simulink model "projekt2"  (R2015a)
settings: Solver=ode3  StartTime=0.0  StopTime=100.0  FixedStep=0.001  RelTol=1e-3
libraries: powerlib_meascontrol x3, simulink_extras x3, sldrtlib x1
settings Model: NumberOfSteps=1000  Creator=Michał  LastModifiedBy=Piotr
settings DebuggingCC: SFNoUnconditionalDefaultTransitionDiag=none

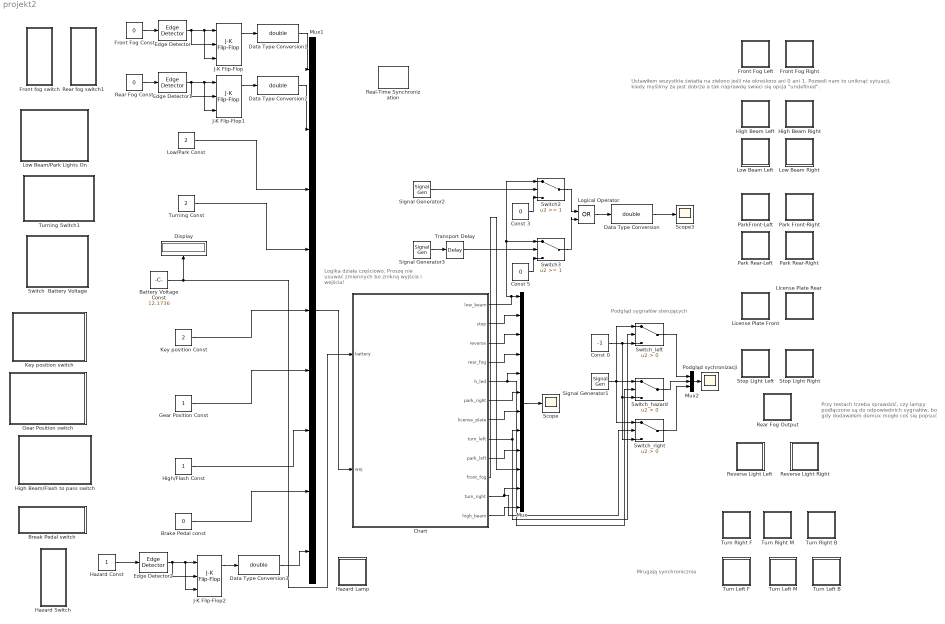
== system projekt2 ==
  note: Mrugają synchronicznie
  note: Przy testach trzeba sprawdzić,
      | czy lampy podłączone są do
      | odpowiednich sygnałów, bo gdy
      | dodawałem demux mogło coś się popsuć
  note: Logika działa częściowo.
      | Proszę nie usuwać zmiennych bo
      |  znikną wyjścia i wejścia!
  note: Podgląd sygnałów sterujących
  note: Ustawiłem wszystkie światła na zielono jeśli nie określono ani 0 ani 1.
      | Pozwoli nam to uniknąć sytuacji, kiedy myślimy że jest dobrze a tak naprawdę swieci się opcja "undefined".
  Battery Voltage Const : Constant  Value=12.1736
  Brake Pedal const : Constant  Value=0
  Break Pedal switch : Subsystem  DialogController=hmiCreateDDGDialog  IsWebBlock=on  mask(MathWorksWebBlock){webBlockId=9203b425-6a6c-4a56-bfc7-19389e98b110, webBlockType=sliderswitch, ShowInLibBrowser=on, ShowInitialText=on, HMISrcModelName=projekt2_bro}
      mask prompts: webBlockId "WebBlock Id"; webBlockType "WebBlock Type"; HMISrcModelName "Source Model"
      mask Help: helpview([docroot '/mapfiles/simulink.map'], 'hmi_slider_switch')
      mask Display:
      | if strcmp(get_param(bdroot(gcb),'BlockDiagramType'), 'library')
      |     image([(matlabroot) '/toolbox/simulink/hmi/icons/SliderSwitch.png']);
      | end
  Chart : Stateflow chart  TreatAsAtomicUnit=on
  Const 0 : Constant  Value=-1
  Const 3 : Constant  Value=0
  Const 5 : Constant  Value=0
  Data Type Conversion{,1..3} (4 alike) : DataTypeConversion  OutDataTypeStr=double
  Display : Display
  Edge Detector : powerlib_meascontrol/Logic/Edge Detector  model=Rising  ic=0  Ts=0
  Edge Detector1 : powerlib_meascontrol/Logic/Edge Detector  model=Rising  ic=0  Ts=0
  Edge Detector2 : powerlib_meascontrol/Logic/Edge Detector  model=Rising  ic=0  Ts=0
  Front Fog Const : Constant  Value=0
  Front Fog Left : Subsystem  DialogController=hmiCreateDDGDialog  IsWebBlock=on  mask(MathWorksWebBlock){webBlockId=1137b8ce-eb4e-40f8-b4a0-8fd8244cb3ae, webBlockType=lamp, ShowInLibBrowser=on, ShowInitialText=on, HMISrcModelName=projekt2_bro}
      mask prompts: webBlockType "WebBlock Type"; HMISrcModelName "Source Model"
      mask Help: helpview([docroot '/mapfiles/simulink.map'], 'hmi_lamp')
      mask Display:
      | if strcmp(get_param(bdroot(gcb),'BlockDiagramType'), 'library')
      |     image([(matlabroot) '/toolbox/simulink/hmi/icons/Lamp.png']);
      | end
  Front Fog Right : Subsystem  DialogController=hmiCreateDDGDialog  IsWebBlock=on  mask(MathWorksWebBlock){webBlockId=91a87ca5-cdac-4de7-a024-86dcea0ba100, webBlockType=lamp, ShowInLibBrowser=on, ShowInitialText=on, HMISrcModelName=projekt2_bro}
      mask prompts: webBlockType "WebBlock Type"; HMISrcModelName "Source Model"
      mask Help: helpview([docroot '/mapfiles/simulink.map'], 'hmi_lamp')
      mask Display:
      | if strcmp(get_param(bdroot(gcb),'BlockDiagramType'), 'library')
      |     image([(matlabroot) '/toolbox/simulink/hmi/icons/Lamp.png']);
      | end
  Front fog switch : Subsystem  DialogController=hmiCreateDDGDialog  IsWebBlock=on  mask(MathWorksWebBlock){webBlockId=82ea03f9-1116-4696-a3c0-68725e62bad1, webBlockType=toggleswitch, ShowInLibBrowser=on, ShowInitialText=on, HMISrcModelName=projekt2_bro}
      mask prompts: webBlockId "WebBlock Id"; webBlockType "WebBlock Type"; HMISrcModelName "Source Model"
      mask Help: helpview([docroot '/mapfiles/simulink.map'], 'hmi_toggle_switch')
      mask Display:
      | if strcmp(get_param(bdroot(gcb),'BlockDiagramType'), 'library')
      |     image([(matlabroot) '/toolbox/simulink/hmi/icons/ToggleSwitch.png']);
      | end
  Gear Position Const : Constant
  Gear Position switch : Subsystem  DialogController=hmiCreateDDGDialog  IsWebBlock=on  mask(MathWorksWebBlock){webBlockId=9873bca9-f904-40ed-a9f4-ca11686aee94, webBlockType=discreteknob, ShowInLibBrowser=on, ShowInitialText=on, HMISrcModelName=projekt2_bro}
      mask prompts: webBlockId "WebBlock Id"; webBlockType "WebBlock Type"; HMISrcModelName "Source Model"
      mask Help: helpview([docroot '/mapfiles/simulink.map'], 'hmi_rotary_switch')
      mask Display:
      | model = bdroot(gcb);
      | if strcmp(get_param(model,'BlockDiagramType'), 'library')
      |     image([(matlabroot) '/toolbox/simulink/hmi/icons/DiscreteKnob.png']);
      | end
  Hazard Const : Constant
  Hazard Lamp : Subsystem  DialogController=hmiCreateDDGDialog  IsWebBlock=on  mask(MathWorksWebBlock){webBlockId=bb1142b6-d357-4f8e-bbaa-be8425e77c63, webBlockType=lamp, ShowInLibBrowser=on, ShowInitialText=on, HMISrcModelName=projekt2_bro}
      mask prompts: webBlockType "WebBlock Type"; HMISrcModelName "Source Model"
      mask Help: helpview([docroot '/mapfiles/simulink.map'], 'hmi_lamp')
      mask Display:
      | if strcmp(get_param(bdroot(gcb),'BlockDiagramType'), 'library')
      |     image([(matlabroot) '/toolbox/simulink/hmi/icons/Lamp.png']);
      | end
  Hazard Switch : Subsystem  DialogController=hmiCreateDDGDialog  IsWebBlock=on  mask(MathWorksWebBlock){webBlockId=797843e7-9493-43d7-b5ed-a5b1ec2f2620, webBlockType=toggleswitch, ShowInLibBrowser=on, ShowInitialText=on, HMISrcModelName=projekt2_bro}
      mask prompts: webBlockId "WebBlock Id"; webBlockType "WebBlock Type"; HMISrcModelName "Source Model"
      mask Help: helpview([docroot '/mapfiles/simulink.map'], 'hmi_toggle_switch')
      mask Display:
      | if strcmp(get_param(bdroot(gcb),'BlockDiagramType'), 'library')
      |     image([(matlabroot) '/toolbox/simulink/hmi/icons/ToggleSwitch.png']);
      | end
  High Beam Left : Subsystem  DialogController=hmiCreateDDGDialog  IsWebBlock=on  mask(MathWorksWebBlock){webBlockId=ca8d7307-15bb-4202-84d0-933cf6b75606, webBlockType=lamp, ShowInLibBrowser=on, ShowInitialText=on, HMISrcModelName=projekt2_bro}
      mask prompts: webBlockType "WebBlock Type"; HMISrcModelName "Source Model"
      mask Help: helpview([docroot '/mapfiles/simulink.map'], 'hmi_lamp')
      mask Display:
      | if strcmp(get_param(bdroot(gcb),'BlockDiagramType'), 'library')
      |     image([(matlabroot) '/toolbox/simulink/hmi/icons/Lamp.png']);
      | end
  High Beam Right : Subsystem  DialogController=hmiCreateDDGDialog  IsWebBlock=on  mask(MathWorksWebBlock){webBlockId=1f4769ad-4ae1-430d-b7b3-b710370c0a18, webBlockType=lamp, ShowInLibBrowser=on, ShowInitialText=on, HMISrcModelName=projekt2_bro}
      mask prompts: webBlockType "WebBlock Type"; HMISrcModelName "Source Model"
      mask Help: helpview([docroot '/mapfiles/simulink.map'], 'hmi_lamp')
      mask Display:
      | if strcmp(get_param(bdroot(gcb),'BlockDiagramType'), 'library')
      |     image([(matlabroot) '/toolbox/simulink/hmi/icons/Lamp.png']);
      | end
  High Beam/Flash to pass switch : Subsystem  DialogController=hmiCreateDDGDialog  IsWebBlock=on  mask(MathWorksWebBlock){webBlockId=cb76618a-e943-4ab4-b6d9-c65f6536b605, webBlockType=discreteknob, ShowInLibBrowser=on, ShowInitialText=on, HMISrcModelName=projekt2_bro}
      mask prompts: webBlockId "WebBlock Id"; webBlockType "WebBlock Type"; HMISrcModelName "Source Model"
      mask Help: helpview([docroot '/mapfiles/simulink.map'], 'hmi_rotary_switch')
      mask Display:
      | model = bdroot(gcb);
      | if strcmp(get_param(model,'BlockDiagramType'), 'library')
      |     image([(matlabroot) '/toolbox/simulink/hmi/icons/DiscreteKnob.png']);
      | end
  High/Flash Const : Constant
  J-K Flip-Flop : simulink_extras/Flip Flops/J-K Flip-Flop  initial_condition=0
  J-K Flip-Flop1 : simulink_extras/Flip Flops/J-K Flip-Flop  initial_condition=0
  J-K Flip-Flop2 : simulink_extras/Flip Flops/J-K Flip-Flop  initial_condition=0
  Key position Const : Constant  Value=2
  Key position switch : Subsystem  DialogController=hmiCreateDDGDialog  IsWebBlock=on  mask(MathWorksWebBlock){webBlockId=6a93fa06-9241-43a4-9533-b6adabf72aa1, webBlockType=discreteknob, ShowInLibBrowser=on, ShowInitialText=on, HMISrcModelName=projekt2_bro}
      mask prompts: webBlockId "WebBlock Id"; webBlockType "WebBlock Type"; HMISrcModelName "Source Model"
      mask Help: helpview([docroot '/mapfiles/simulink.map'], 'hmi_rotary_switch')
      mask Display:
      | model = bdroot(gcb);
      | if strcmp(get_param(model,'BlockDiagramType'), 'library')
      |     image([(matlabroot) '/toolbox/simulink/hmi/icons/DiscreteKnob.png']);
      | end
  License Plate Front : Subsystem  DialogController=hmiCreateDDGDialog  IsWebBlock=on  mask(MathWorksWebBlock){webBlockId=33e809d7-7293-40ab-82d3-89bf48253b8e, webBlockType=lamp, ShowInLibBrowser=on, ShowInitialText=on, HMISrcModelName=projekt2_bro}
      mask prompts: webBlockType "WebBlock Type"; HMISrcModelName "Source Model"
      mask Help: helpview([docroot '/mapfiles/simulink.map'], 'hmi_lamp')
      mask Display:
      | if strcmp(get_param(bdroot(gcb),'BlockDiagramType'), 'library')
      |     image([(matlabroot) '/toolbox/simulink/hmi/icons/Lamp.png']);
      | end
  License Plate Rear : Subsystem  DialogController=hmiCreateDDGDialog  IsWebBlock=on  mask(MathWorksWebBlock){webBlockId=e2d37614-ade8-4960-9755-81aca5d14707, webBlockType=lamp, ShowInLibBrowser=on, ShowInitialText=on, HMISrcModelName=projekt2_bro}
      mask prompts: webBlockType "WebBlock Type"; HMISrcModelName "Source Model"
      mask Help: helpview([docroot '/mapfiles/simulink.map'], 'hmi_lamp')
      mask Display:
      | if strcmp(get_param(bdroot(gcb),'BlockDiagramType'), 'library')
      |     image([(matlabroot) '/toolbox/simulink/hmi/icons/Lamp.png']);
      | end
  Logical Operator : Logic  Operator=OR  IconShape=distinctive  AllPortsSameDT=off  OutDataTypeStr=boolean
  Low Beam Left : Subsystem  DialogController=hmiCreateDDGDialog  IsWebBlock=on  mask(MathWorksWebBlock){webBlockId=93f46513-60d2-4d66-bc1a-d0f0cd962895, webBlockType=lamp, ShowInLibBrowser=on, ShowInitialText=on, HMISrcModelName=projekt2_bro}
      mask prompts: webBlockType "WebBlock Type"; HMISrcModelName "Source Model"
      mask Help: helpview([docroot '/mapfiles/simulink.map'], 'hmi_lamp')
      mask Display:
      | if strcmp(get_param(bdroot(gcb),'BlockDiagramType'), 'library')
      |     image([(matlabroot) '/toolbox/simulink/hmi/icons/Lamp.png']);
      | end
  Low Beam Right : Subsystem  DialogController=hmiCreateDDGDialog  IsWebBlock=on  mask(MathWorksWebBlock){webBlockId=cbd13759-b6c8-48cc-8b95-5d08102353a4, webBlockType=lamp, ShowInLibBrowser=on, ShowInitialText=on, HMISrcModelName=projekt2_bro}
      mask prompts: webBlockType "WebBlock Type"; HMISrcModelName "Source Model"
      mask Help: helpview([docroot '/mapfiles/simulink.map'], 'hmi_lamp')
      mask Display:
      | if strcmp(get_param(bdroot(gcb),'BlockDiagramType'), 'library')
      |     image([(matlabroot) '/toolbox/simulink/hmi/icons/Lamp.png']);
      | end
  Low Beam/Park Lights On : Subsystem  DialogController=hmiCreateDDGDialog  IsWebBlock=on  mask(MathWorksWebBlock){webBlockId=c2ad75a2-8b3b-4bc8-8975-68c2dc12f70e, webBlockType=discreteknob, ShowInLibBrowser=on, ShowInitialText=on, HMISrcModelName=projekt2_bro}
      mask prompts: webBlockId "WebBlock Id"; webBlockType "WebBlock Type"; HMISrcModelName "Source Model"
      mask Help: helpview([docroot '/mapfiles/simulink.map'], 'hmi_rotary_switch')
      mask Display:
      | model = bdroot(gcb);
      | if strcmp(get_param(model,'BlockDiagramType'), 'library')
      |     image([(matlabroot) '/toolbox/simulink/hmi/icons/DiscreteKnob.png']);
      | end
  Low/Park Const : Constant  Value=2
  Mux : Mux  Inputs=12
  Mux1 : Mux  Inputs=9
  Mux2 : Mux  Inputs=3
  Park Front-Right : Subsystem  DialogController=hmiCreateDDGDialog  IsWebBlock=on  mask(MathWorksWebBlock){webBlockId=9b7f9617-a09f-4c99-8fef-94e297c97476, webBlockType=lamp, ShowInLibBrowser=on, ShowInitialText=on, HMISrcModelName=projekt2_bro}
      mask prompts: webBlockType "WebBlock Type"; HMISrcModelName "Source Model"
      mask Help: helpview([docroot '/mapfiles/simulink.map'], 'hmi_lamp')
      mask Display:
      | if strcmp(get_param(bdroot(gcb),'BlockDiagramType'), 'library')
      |     image([(matlabroot) '/toolbox/simulink/hmi/icons/Lamp.png']);
      | end
  Park Rear-Left : Subsystem  DialogController=hmiCreateDDGDialog  IsWebBlock=on  mask(MathWorksWebBlock){webBlockId=f0d072a0-1d13-4b2c-9055-2934ad2aeeda, webBlockType=lamp, ShowInLibBrowser=on, ShowInitialText=on, HMISrcModelName=projekt2_bro}
      mask prompts: webBlockType "WebBlock Type"; HMISrcModelName "Source Model"
      mask Help: helpview([docroot '/mapfiles/simulink.map'], 'hmi_lamp')
      mask Display:
      | if strcmp(get_param(bdroot(gcb),'BlockDiagramType'), 'library')
      |     image([(matlabroot) '/toolbox/simulink/hmi/icons/Lamp.png']);
      | end
  Park Rear-Right : Subsystem  DialogController=hmiCreateDDGDialog  IsWebBlock=on  mask(MathWorksWebBlock){webBlockId=6a2c4c4f-cbef-489d-a936-82416b980595, webBlockType=lamp, ShowInLibBrowser=on, ShowInitialText=on, HMISrcModelName=projekt2_bro}
      mask prompts: webBlockType "WebBlock Type"; HMISrcModelName "Source Model"
      mask Help: helpview([docroot '/mapfiles/simulink.map'], 'hmi_lamp')
      mask Display:
      | if strcmp(get_param(bdroot(gcb),'BlockDiagramType'), 'library')
      |     image([(matlabroot) '/toolbox/simulink/hmi/icons/Lamp.png']);
      | end
  ParkFront-Left : Subsystem  DialogController=hmiCreateDDGDialog  IsWebBlock=on  mask(MathWorksWebBlock){webBlockId=2a1e2c86-b327-4131-a799-a6f04c855dbb, webBlockType=lamp, ShowInLibBrowser=on, ShowInitialText=on, HMISrcModelName=projekt2_bro}
      mask prompts: webBlockType "WebBlock Type"; HMISrcModelName "Source Model"
      mask Help: helpview([docroot '/mapfiles/simulink.map'], 'hmi_lamp')
      mask Display:
      | if strcmp(get_param(bdroot(gcb),'BlockDiagramType'), 'library')
      |     image([(matlabroot) '/toolbox/simulink/hmi/icons/Lamp.png']);
      | end
  Podgląd sychronizacji : Scope
  Real-Time Synchronization : sldrtlib/Real-Time Synchronization  SampleTime=0.1  MaxMissedTicks=10  ShowMissedTicks=off  YieldWhenWaiting=off
  Rear Fog Const : Constant  Value=0
  Rear Fog Output : Subsystem  DialogController=hmiCreateDDGDialog  IsWebBlock=on  mask(MathWorksWebBlock){webBlockId=c86d492b-d5b5-45fd-8d57-4ca5ff4cc7e3, webBlockType=lamp, ShowInLibBrowser=on, ShowInitialText=on, HMISrcModelName=projekt2_bro}
      mask prompts: webBlockType "WebBlock Type"; HMISrcModelName "Source Model"
      mask Help: helpview([docroot '/mapfiles/simulink.map'], 'hmi_lamp')
      mask Display:
      | if strcmp(get_param(bdroot(gcb),'BlockDiagramType'), 'library')
      |     image([(matlabroot) '/toolbox/simulink/hmi/icons/Lamp.png']);
      | end
  Rear fog switch1 : Subsystem  DialogController=hmiCreateDDGDialog  IsWebBlock=on  mask(MathWorksWebBlock){webBlockId=a6fd6b9e-e7fc-4e66-962f-fca6c1e6a3ec, webBlockType=toggleswitch, ShowInLibBrowser=on, ShowInitialText=on, HMISrcModelName=projekt2_bro}
      mask prompts: webBlockId "WebBlock Id"; webBlockType "WebBlock Type"; HMISrcModelName "Source Model"
      mask Help: helpview([docroot '/mapfiles/simulink.map'], 'hmi_toggle_switch')
      mask Display:
      | if strcmp(get_param(bdroot(gcb),'BlockDiagramType'), 'library')
      |     image([(matlabroot) '/toolbox/simulink/hmi/icons/ToggleSwitch.png']);
      | end
  Reverse Light Left : Subsystem  DialogController=hmiCreateDDGDialog  IsWebBlock=on  mask(MathWorksWebBlock){webBlockId=1216e6e6-a2b0-45d0-bfe3-2d719345f04b, webBlockType=lamp, ShowInLibBrowser=on, ShowInitialText=on, HMISrcModelName=projekt2_bro}
      mask prompts: webBlockType "WebBlock Type"; HMISrcModelName "Source Model"
      mask Help: helpview([docroot '/mapfiles/simulink.map'], 'hmi_lamp')
      mask Display:
      | if strcmp(get_param(bdroot(gcb),'BlockDiagramType'), 'library')
      |     image([(matlabroot) '/toolbox/simulink/hmi/icons/Lamp.png']);
      | end
  Reverse Light Right : Subsystem  DialogController=hmiCreateDDGDialog  IsWebBlock=on  mask(MathWorksWebBlock){webBlockId=aab8cf70-1b34-41c4-b955-76454d5b273c, webBlockType=lamp, ShowInLibBrowser=on, ShowInitialText=on, HMISrcModelName=projekt2_bro}
      mask prompts: webBlockType "WebBlock Type"; HMISrcModelName "Source Model"
      mask Help: helpview([docroot '/mapfiles/simulink.map'], 'hmi_lamp')
      mask Display:
      | if strcmp(get_param(bdroot(gcb),'BlockDiagramType'), 'library')
      |     image([(matlabroot) '/toolbox/simulink/hmi/icons/Lamp.png']);
      | end
  Scope : Scope
  Scope3 : Scope
      settings: SaveName=ScopeData3
  Signal Generator1 : SignalGenerator  WaveForm=square  Frequency=1.5
  Signal Generator2 : SignalGenerator  WaveForm=square  Frequency=100
  Signal Generator3 : SignalGenerator  WaveForm=square  Frequency=100
  Stop Light Left : Subsystem  DialogController=hmiCreateDDGDialog  IsWebBlock=on  mask(MathWorksWebBlock){webBlockId=fe2cd1c8-1e5b-41df-9169-199d59002129, webBlockType=lamp, ShowInLibBrowser=on, ShowInitialText=on, HMISrcModelName=projekt2_bro}
      mask prompts: webBlockType "WebBlock Type"; HMISrcModelName "Source Model"
      mask Help: helpview([docroot '/mapfiles/simulink.map'], 'hmi_lamp')
      mask Display:
      | if strcmp(get_param(bdroot(gcb),'BlockDiagramType'), 'library')
      |     image([(matlabroot) '/toolbox/simulink/hmi/icons/Lamp.png']);
      | end
  Stop Light Right : Subsystem  DialogController=hmiCreateDDGDialog  IsWebBlock=on  mask(MathWorksWebBlock){webBlockId=e28d537a-d055-4b98-9d36-b585e9c6a455, webBlockType=lamp, ShowInLibBrowser=on, ShowInitialText=on, HMISrcModelName=projekt2_bro}
      mask prompts: webBlockType "WebBlock Type"; HMISrcModelName "Source Model"
      mask Help: helpview([docroot '/mapfiles/simulink.map'], 'hmi_lamp')
      mask Display:
      | if strcmp(get_param(bdroot(gcb),'BlockDiagramType'), 'library')
      |     image([(matlabroot) '/toolbox/simulink/hmi/icons/Lamp.png']);
      | end
  Switch  Battery Voltage : Subsystem  DialogController=hmiCreateDDGDialog  IsWebBlock=on  mask(MathWorksWebBlock){webBlockId=9fcb4338-6d0a-49e3-9d35-1b064d171cad, webBlockType=continuousknob, ShowInLibBrowser=on, ShowInitialText=on, HMISrcModelName=projekt2_bro}
      mask prompts: webBlockId "WebBlock Id"; webBlockType "WebBlock Type"; HMISrcModelName "Source Model"
      mask Help: helpview([docroot '/mapfiles/simulink.map'], 'hmi_knob')
      mask Display:
      | if strcmp(get_param(bdroot(gcb),'BlockDiagramType'), 'library')
      |     image([(matlabroot) '/toolbox/simulink/hmi/icons/ContinuousKnob.png']);
      | end
  Switch2 : Switch  Threshold=1
  Switch3 : Switch  Threshold=1
  Switch_hazard : Switch  Criteria=u2 > Threshold
  Switch_left : Switch  Criteria=u2 > Threshold
  Switch_right : Switch  Criteria=u2 > Threshold
  Transport Delay : TransportDelay  DelayTime=0.004
  Turn Left B : Subsystem  DialogController=hmiCreateDDGDialog  IsWebBlock=on  mask(MathWorksWebBlock){webBlockId=4dada64b-7e7a-4b74-8d0d-b8c062fae480, webBlockType=lamp, ShowInLibBrowser=on, ShowInitialText=on, HMISrcModelName=projekt2_bro}
      mask prompts: webBlockType "WebBlock Type"; HMISrcModelName "Source Model"
      mask Help: helpview([docroot '/mapfiles/simulink.map'], 'hmi_lamp')
      mask Display:
      | if strcmp(get_param(bdroot(gcb),'BlockDiagramType'), 'library')
      |     image([(matlabroot) '/toolbox/simulink/hmi/icons/Lamp.png']);
      | end
  Turn Left F : Subsystem  DialogController=hmiCreateDDGDialog  IsWebBlock=on  mask(MathWorksWebBlock){webBlockId=e6f60506-cdc4-4a96-ad0a-e579d3159bd8, webBlockType=lamp, ShowInLibBrowser=on, ShowInitialText=on, HMISrcModelName=projekt2_bro}
      mask prompts: webBlockType "WebBlock Type"; HMISrcModelName "Source Model"
      mask Help: helpview([docroot '/mapfiles/simulink.map'], 'hmi_lamp')
      mask Display:
      | if strcmp(get_param(bdroot(gcb),'BlockDiagramType'), 'library')
      |     image([(matlabroot) '/toolbox/simulink/hmi/icons/Lamp.png']);
      | end
  Turn Left M : Subsystem  DialogController=hmiCreateDDGDialog  IsWebBlock=on  mask(MathWorksWebBlock){webBlockId=86cbbfda-27e6-47d5-9477-a59dd7b37ef2, webBlockType=lamp, ShowInLibBrowser=on, ShowInitialText=on, HMISrcModelName=projekt2_bro}
      mask prompts: webBlockType "WebBlock Type"; HMISrcModelName "Source Model"
      mask Help: helpview([docroot '/mapfiles/simulink.map'], 'hmi_lamp')
      mask Display:
      | if strcmp(get_param(bdroot(gcb),'BlockDiagramType'), 'library')
      |     image([(matlabroot) '/toolbox/simulink/hmi/icons/Lamp.png']);
      | end
  Turn Right B : Subsystem  DialogController=hmiCreateDDGDialog  IsWebBlock=on  mask(MathWorksWebBlock){webBlockId=de10194a-7102-4529-bffa-3ba9fd236063, webBlockType=lamp, ShowInLibBrowser=on, ShowInitialText=on, HMISrcModelName=projekt2_bro}
      mask prompts: webBlockType "WebBlock Type"; HMISrcModelName "Source Model"
      mask Help: helpview([docroot '/mapfiles/simulink.map'], 'hmi_lamp')
      mask Display:
      | if strcmp(get_param(bdroot(gcb),'BlockDiagramType'), 'library')
      |     image([(matlabroot) '/toolbox/simulink/hmi/icons/Lamp.png']);
      | end
  Turn Right F : Subsystem  DialogController=hmiCreateDDGDialog  IsWebBlock=on  mask(MathWorksWebBlock){webBlockId=8d34aea4-920d-4358-901e-989a77b658ef, webBlockType=lamp, ShowInLibBrowser=on, ShowInitialText=on, HMISrcModelName=projekt2_bro}
      mask prompts: webBlockType "WebBlock Type"; HMISrcModelName "Source Model"
      mask Help: helpview([docroot '/mapfiles/simulink.map'], 'hmi_lamp')
      mask Display:
      | if strcmp(get_param(bdroot(gcb),'BlockDiagramType'), 'library')
      |     image([(matlabroot) '/toolbox/simulink/hmi/icons/Lamp.png']);
      | end
  Turn Right M : Subsystem  DialogController=hmiCreateDDGDialog  IsWebBlock=on  mask(MathWorksWebBlock){webBlockId=1d267936-957d-42ac-8213-13ca1cae1405, webBlockType=lamp, ShowInLibBrowser=on, ShowInitialText=on, HMISrcModelName=projekt2_bro}
      mask prompts: webBlockType "WebBlock Type"; HMISrcModelName "Source Model"
      mask Help: helpview([docroot '/mapfiles/simulink.map'], 'hmi_lamp')
      mask Display:
      | if strcmp(get_param(bdroot(gcb),'BlockDiagramType'), 'library')
      |     image([(matlabroot) '/toolbox/simulink/hmi/icons/Lamp.png']);
      | end
  Turning Const : Constant  Value=2
  Turning Switch1 : Subsystem  DialogController=hmiCreateDDGDialog  IsWebBlock=on  mask(MathWorksWebBlock){webBlockId=0fc1dd6b-b7af-4fe7-8c63-8dd4046cb8f2, webBlockType=discreteknob, ShowInLibBrowser=on, ShowInitialText=on, HMISrcModelName=projekt2_bro}
      mask prompts: webBlockId "WebBlock Id"; webBlockType "WebBlock Type"; HMISrcModelName "Source Model"
      mask Help: helpview([docroot '/mapfiles/simulink.map'], 'hmi_rotary_switch')
      mask Display:
      | model = bdroot(gcb);
      | if strcmp(get_param(model,'BlockDiagramType'), 'library')
      |     image([(matlabroot) '/toolbox/simulink/hmi/icons/DiscreteKnob.png']);
      | end
  wires:
  Battery Voltage Const/1 -> Chart/1(battery), Display/1
  Chart/1(low_beam) -> Mux/1, Switch3/1, Switch2/1
  Chart/2(stop) -> Mux/2
  Chart/3(reverse) -> Mux/3
  Chart/4(rear_fog) -> Mux/4
  Chart/6(park_right) -> Mux/6
  Chart/8(turn_left) -> Mux/8, Switch_left/2
  Chart/9(park_left) -> Mux/9
  Chart/10(front_fog) -> Mux/10
  Chart/12(high_beam) -> Mux/12
  Mux/1 -> Scope/1
  Chart/5(h_led) -> Switch_hazard/2, Mux/5
  Low/Park Const/1 -> Mux1/3
  Turning Const/1 -> Mux1/4
  Key position Const/1 -> Mux1/5
  Gear Position Const/1 -> Mux1/6
  High/Flash Const/1 -> Mux1/7
  Brake Pedal const/1 -> Mux1/8
  Mux1/1 -> Chart/2(wej)
  Chart/7(license_plate) -> Mux/7
  Chart/11(turn_right) -> Mux/11, Switch_right/2
  Switch_left/1 -> Mux2/1
  Const 0/1 -> Switch_right/3, Switch_hazard/3, Switch_left/3
  Switch_right/1 -> Mux2/3
  Signal Generator1/1 -> Switch_hazard/1, Switch_right/1, Switch_left/1
  Signal Generator3/1 -> Transport Delay/1
  Data Type Conversion/1 -> Scope3/1
  Signal Generator2/1 -> Switch2/2
  Const 3/1 -> Switch2/3
  Transport Delay/1 -> Switch3/2
  Const 5/1 -> Switch3/3
  Switch3/1 -> Logical Operator/2
  Switch2/1 -> Logical Operator/1
  Logical Operator/1 -> Data Type Conversion/1
  Switch_hazard/1 -> Mux2/2
  Mux2/1 -> Podgląd sychronizacji/1
  Front Fog Const/1 -> Edge Detector/1
  J-K Flip-Flop/1 -> Data Type Conversion1/1
  Data Type Conversion1/1 -> Mux1/1
  Edge Detector/1 -> J-K Flip-Flop/2, J-K Flip-Flop/3, J-K Flip-Flop/1
  J-K Flip-Flop1/1 -> Data Type Conversion2/1
  Edge Detector1/1 -> J-K Flip-Flop1/2, J-K Flip-Flop1/3, J-K Flip-Flop1/1
  Rear Fog Const/1 -> Edge Detector1/1
  Data Type Conversion2/1 -> Mux1/2
  J-K Flip-Flop2/1 -> Data Type Conversion3/1
  Edge Detector2/1 -> J-K Flip-Flop2/2, J-K Flip-Flop2/3, J-K Flip-Flop2/1
  Hazard Const/1 -> Edge Detector2/1
  Data Type Conversion3/1 -> Mux1/9

== system projekt2/Break Pedal switch ==

== system projekt2/Front Fog Left ==

== system projekt2/Front Fog Right ==

== system projekt2/Front fog switch ==

== system projekt2/Gear Position switch ==

== system projekt2/Hazard Lamp ==

== system projekt2/Hazard Switch ==

== system projekt2/High Beam Left ==

== system projekt2/High Beam Right ==

== system projekt2/High Beam//Flash to pass switch ==

== system projekt2/Key position switch ==

== system projekt2/License Plate Front ==

== system projekt2/License Plate Rear ==

== system projekt2/Low Beam Left ==

== system projekt2/Low Beam Right ==

== system projekt2/Low Beam//Park Lights On ==

== system projekt2/Park Front-Right ==

== system projekt2/Park Rear-Left ==

== system projekt2/Park Rear-Right ==

== system projekt2/ParkFront-Left ==

== system projekt2/Rear Fog Output ==

== system projekt2/Rear fog switch1 ==

== system projekt2/Reverse Light Left ==

== system projekt2/Reverse Light Right ==

== system projekt2/Stop Light Left ==

== system projekt2/Stop Light Right ==

== system projekt2/Switch  Battery Voltage ==

== system projekt2/Turn Left B ==

== system projekt2/Turn Left F ==

== system projekt2/Turn Left M ==

== system projekt2/Turn Right B ==

== system projekt2/Turn Right F ==

== system projekt2/Turn Right M ==

== system projekt2/Turning Switch1 ==

== stateflow chart projekt2/Chart ==
  settings: executeAtInitialization=1  initializeOutput=1
  state battery_good
    state stop [parallel]
      settings: executionOrder=1
      state Stop_lights_on
        entry: stop = 1;
      state Stop_lights_off
        entry: stop = 0;
      Stop_lights_off -> Stop_lights_on : [wej(8) == 1]
      (default) -> Stop_lights_off
      Stop_lights_on -> Stop_lights_off : [wej(8) == 0]
    state high_beam_and_flash [parallel]
      settings: executionOrder=8
      state high_beam_on
        entry: high_beam = 1;
      state high_beam_off
        entry: high_beam = 0;
      state flash_to_pass_on
        entry: high_beam = 1;
      high_beam_off -> high_beam_on [order 1] : [wej(3) == 1 & wej(7) == 1 & wej(5)==2]
      high_beam_on -> high_beam_off [order 1] : [wej(7) == 0 | wej(5)~=2]
      high_beam_on -> flash_to_pass_on [order 2] : [wej(7) == 2]
      flash_to_pass_on -> high_beam_on [order 2] : [wej(7) == 1 & wej(3) == 1]
      (default) -> high_beam_off
      high_beam_off -> flash_to_pass_on [order 2] : [wej(7) == 2 & wej(5)==2]
      flash_to_pass_on -> high_beam_off [order 1] : [wej(7) == 0 | wej(5)~=2]
    state low_park [parallel]
      settings: executionOrder=2
      state low_beam_on
        entry: low_beam = 1;
        park_left = 1;
        park_right = 1;
      state low_beam_off
        entry: low_beam = 0;
        park_left = 0;
        park_right = 0;
      state park_light_on
        entry: park_left = 1;
        park_right = 1;
        low_beam = 0;
      park_light_on -> low_beam_on [order 2] : [wej(3) == 1]
      low_beam_on -> park_light_on [order 2] : [wej(3) == 2]
      low_beam_off -> low_beam_on [order 2] : [wej(3) == 1]
      (default) -> low_beam_off
      low_beam_on -> low_beam_off [order 1] : [wej(3) == 0]
      park_light_on -> low_beam_off [order 1] : [wej(3) == 0]
      low_beam_off -> park_light_on [order 1] : [wej(3) == 2]
    note: Flash to pass do poprawki
    state reverse [parallel]
      settings: executionOrder=7
      state reverse_off
        entry: reverse = 0;
      state reverse_on
        entry: reverse = 1;
      (default) -> reverse_off
      reverse_off -> reverse_on : [wej(6) == 6 & wej(5)==2]
      reverse_on -> reverse_off : [wej(6) ~= 6 & wej(5)~=2]
    state license_plate [parallel]
      settings: executionOrder=6
      state license_on
        entry:license_plate=1
      state license_off
        entry:license_plate=0
      license_on -> license_off : [wej(3)==0]
      (default) -> license_off
      license_off -> license_on : [wej(3)~=1]
    state front_fog [parallel]
      settings: executionOrder=4
      state front_fog_off
        entry: front_fog = 0;
      state front_fog_on
        entry: front_fog = 1;
      (default) -> front_fog_off
      front_fog_off -> front_fog_on : [wej(1) == 1 & (wej(3) == 1 | wej(3) == 2) & (wej(5)==2 | wej(5)==3)]
      front_fog_on -> front_fog_off : [wej(1) == 0 | wej(3) == 0 | wej(5)==2 | wej(5)==3]
    state rear_fog [parallel]
      settings: executionOrder=5
      state rear_fog_on
        entry: rear_fog = 0;
      state rear_fog_off
        entry: rear_fog = 1;
      (default) -> rear_fog_on
      rear_fog_on -> rear_fog_off : [wej(2) == 1 & wej(3) ==1 & (wej(5)==2 | wej(5)==3)]
      rear_fog_off -> rear_fog_on : [wej(2) == 0 | wej (3) ~= 1 | wej(5)==2 | wej(5)==3]
    state turn [parallel]
      settings: executionOrder=3
      state turn_right_or_left
        entry:h_led=0;
        state turn_left_on1
          entry: turn_left = 1;
          turn_right = 0;
        state turn_off1
          entry: turn_right = 0;
          turn_left = 0;
        state turn_right_on1
          entry: turn_right = 1;
          turn_left = 0;
        turn_off1 -> turn_left_on1 [order 1] : [wej(4) == 0 & (wej(5)==2 | wej(5)==3)]
        turn_left_on1 -> turn_off1 [order 1] : [wej(4) == 1 & (wej(5)==0 | wej(5)==1)]
        (default) -> turn_off1
        turn_right_on1 -> turn_left_on1 [order 1] : [wej(4) == 0]
        turn_left_on1 -> turn_right_on1 [order 2] : [wej(4) == 2]
        turn_off1 -> turn_right_on1 [order 2] : [wej(4) == 2 & (wej(5)==2 | wej(5)==3)]
        turn_right_on1 -> turn_off1 [order 2] : [wej(4) == 1 & (wej(5)==0 | wej(5)==1)]
      state hazard_on
        entry:h_led=1
        entry:turn_left=1
        entry:turn_right=1
      (default) -> turn_right_or_left
      turn_right_or_left -> hazard_on : [wej(9)==1]
      hazard_on -> turn_right_or_left : [wej(9)==0]
  state battery_bad
    entry:h_led=0;
    entry:front_fog = 0;
    entry:high_beam =0;
    entry:low_beam = 0;
    entry:park_left = 0;
    entry:park_right = 0;
    entry:license_plate = 0;
    entry:stop = 0;
    entry:rear_fog = 0;
    entry:reverse = 0;
    entry:turn_left = 0;
    entry:turn_right = 0;
  state battery_error
    entry:h_led=0;
    entry:front_fog = 0;
    entry:high_beam =0;
    entry:low_beam = 0;
    entry:park_left = 0;
    entry:park_right = 0;
    entry:license_plate = 0;
    entry:stop = 0;
    entry:rear_fog = 0;
    entry: reverse = 0;
    entry:turn_left = 0;
    entry:turn_right = 0;
  note: ?
  (default) -> battery_bad
  battery_bad -> battery_good [order 2] : [battery>=6 & battery<=18]
  battery_good -> battery_bad [order 1] : [(battery>=0 & battery<6) | (battery>18 & battery<=26)]
  battery_bad -> battery_error [order 1] : [battery<0 | battery>26]
  battery_good -> battery_error [order 2] : [battery < 0 | battery >26]
  data: battery input; low_beam output; stop output; reverse output; rear_fog output; h_led output; park_right output; license_plate output; turn_left output; park_left output; front_fog output; turn_right output; high_beam output; wej input
